simulink library "HybridFEMLibrary"  (Simulink 7.9)
settings: Solver=ode45  SolverMode=SingleTasking  StartTime=0.0  StopTime=10.0  RelTol=1e-3
values from neighbouring files (symbols this model uses):
  Elements = ElementsBack    [ModelSetup.m]
  Integrator = CreateIntegrator(data(3), data(4), data(5), data(1), data(2))    [LoadConfiguration.m]    (also in MatlabSimulation.m = UpdateAccelerationCR(Integrator, Structure, step); ModelSetup.m = InitializeIntegrator(Integrator, Structure))
  sample = SampleRate/Integrator.Interpolations    [ModelSetup.m]
  SampleRate = Integrator.Timestep    [ModelSetup.m]
  Structure = CalculateMatrices(Structure, Elements, Integrator)    [ModelSetup.m]
undefined symbols (not defined in the file or in its folder): DiscIntNeverNeededParam, MNS
libraries: simulink x2
settings Model: Creator=Tommy  LastModifiedBy=Thomas Marullo

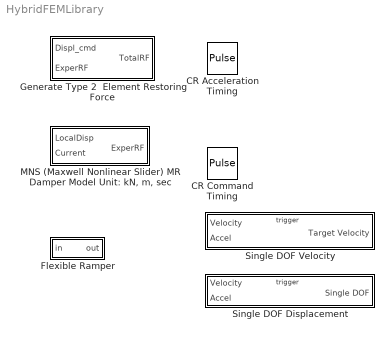
== system HybridFEMLibrary ==
  CR Acceleration Timing : DiscretePulseGenerator  Period=Integrator.Interpolations  PhaseDelay=Integrator.Interpolations-1  SampleTime=sample
  CR Command Timing : DiscretePulseGenerator  Period=Integrator.Interpolations  PulseWidth=Integrator.Interpolations-1  SampleTime=sample
  Flexible Ramper : Subsystem  mask{ramps=Integrator.Interpolations, samplerate=sample, u_old=[0]}
      mask prompts: ramps "Total ramp steps"; samplerate "Sample rate"; u_old "Dimensions"
      mask help:
      | Signal ramper that starts when it detects a change in the current and previous signal. It then ramps for the designated steps and goes back to detecting changes to start ramping again.
      |
      | Set the total number of ramping steps it should interpolate between the current and previous signals.  This will disregard any signal changes for the number of steps desginated.
      | Sample rate should be the sample rate of the system.
      | The source signal sample rate should be the sample rate * total ramp steps to get the best performance.  Otherwise, having a number of ramps smaller than the number of steps between signal changes will result in flat-lining.  Larger ramps than the number of steps between signal changes will result in missed data and poor ramping.
      |
      | Set Dimension variable to an empty array of required size, ie. [0;0;0] for 3 dimensions.
      mask Display:
      | fprintf('%d',ramps)
      | port_label('input',1,'>')
      | port_label('output',1,'>')
  Generate Type 2  Element Restoring Force : Subsystem  mask(Generate Type 2 Element Restoring Force){id=0, simulation=off}
      mask prompts: id "Element ID"; simulation "Experiment Mode"
      mask help:
      | Generates the Restoring Force vector for a Type 2 Element
      |
      | Enter the ID for this element corresponding with the input configuration file.
      |
      | For Simulation mode, uncheck the "Experiment Mode" box.
      | Connect the 'Target Displacement' command from the Integrator to the 'Disp' input.  'ExperRF' is not used with Simulation Mode.
      |
      | For Experiment mode, check the "Experiment Mode" box to activate the Experimental Restoring Force (ExperRF) input.
      | Connect an Experimental Restoring Force feedback (physical or numerical) to the 'ExperRF' input.  The 'Disp' is not used with Experiment mode.
      |
      | Connect the 'TotalRF' output to the 'TotalRF' input of the Integrator block or through a summer block with other Element 'TotalRF' outputs.
      mask Display:
      | disp(id);
      | port_label('input',1,'Disp');
      | port_label('input',2,'ExperRF');
      | port_label('output',1,'TotalRF');
  "MNS (Maxwell Nonlinear Slider) MR Damper Model Unit: kN, m, sec" : Subsystem
      mask Type: MNS MR Damper Model
      mask Description:
      | Used in the local coordinate system, this model requires a Local Displacement from a "Generate Experimental Command" block and feeds the output force to a Type 2 Experimental Element to convert back to global coordinates.
      | 
      | Requires the HybridFEM/scripts/MNS_model_parameters.m file
  Single DOF Displacement : Subsystem  SystemSampleTime=SampleRate  mask{DOF=Elements{1}.Nodes(1).UX}
      mask prompts: DOF "Element DOF"
  Single DOF Velocity : Subsystem  SystemSampleTime=SampleRate  mask{DOF=Elements{1}.Nodes(1).UX}

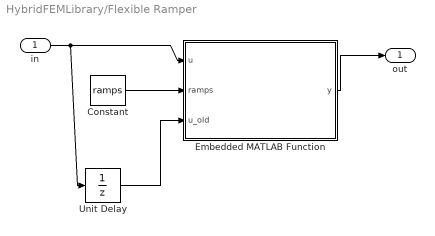
== system HybridFEMLibrary/Flexible Ramper ==
  in : Inport
  Constant : Constant  Value=ramps  SampleTime=samplerate
  Embedded MATLAB Function : MATLAB Function  TreatAsAtomicUnit=on
  Unit Delay : UnitDelay  SampleTime=-1
  out : Outport
  wires:
  in/1 -> Unit Delay/1, Embedded MATLAB Function/1(u)
  Constant/1 -> Embedded MATLAB Function/2(ramps)
  Embedded MATLAB Function/1(y) -> out/1
  Unit Delay/1 -> Embedded MATLAB Function/3(u_old)

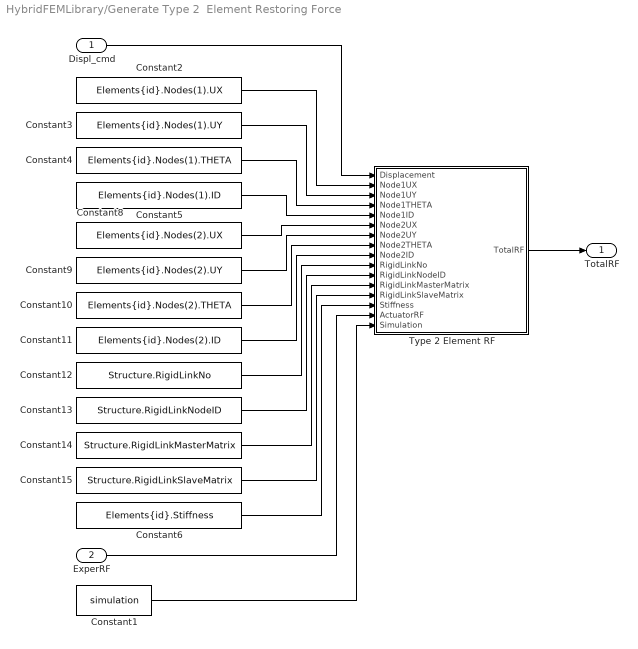
== system HybridFEMLibrary/Generate Type 2  Element Restoring Force ==
  Displ_cmd : Inport
  ExperRF : Inport  Port=2
  Constant1 : Constant  Value=simulation
  Constant10 : Constant  Value=Elements{id}.Nodes(2).THETA
  Constant11 : Constant  Value=Elements{id}.Nodes(2).ID
  Constant12 : Constant  Value=Structure.RigidLinkNo
  Constant13 : Constant  Value=Structure.RigidLinkNodeID
  Constant14 : Constant  Value=Structure.RigidLinkMasterMatrix
  Constant15 : Constant  Value=Structure.RigidLinkSlaveMatrix
  Constant2 : Constant  Value=Elements{id}.Nodes(1).UX
  Constant3 : Constant  Value=Elements{id}.Nodes(1).UY
  Constant4 : Constant  Value=Elements{id}.Nodes(1).THETA
  Constant5 : Constant  Value=Elements{id}.Nodes(1).ID
  Constant6 : Constant  Value=Elements{id}.Stiffness
  Constant8 : Constant  Value=Elements{id}.Nodes(2).UX
  Constant9 : Constant  Value=Elements{id}.Nodes(2).UY
  Type 2 Element RF : MATLAB Function  TreatAsAtomicUnit=on
  TotalRF : Outport
  wires:
  Type 2 Element RF/1(TotalRF) -> TotalRF/1
  Displ_cmd/1 -> Type 2 Element RF/1(Displacement)
  Constant2/1 -> Type 2 Element RF/2(Node1UX)
  Constant3/1 -> Type 2 Element RF/3(Node1UY)
  Constant4/1 -> Type 2 Element RF/4(Node1THETA)
  Constant5/1 -> Type 2 Element RF/5(Node1ID)
  Constant8/1 -> Type 2 Element RF/6(Node2UX)
  Constant9/1 -> Type 2 Element RF/7(Node2UY)
  Constant10/1 -> Type 2 Element RF/8(Node2THETA)
  Constant11/1 -> Type 2 Element RF/9(Node2ID)
  Constant12/1 -> Type 2 Element RF/10(RigidLinkNo)
  Constant13/1 -> Type 2 Element RF/11(RigidLinkNodeID)
  Constant14/1 -> Type 2 Element RF/12(RigidLinkMasterMatrix)
  Constant15/1 -> Type 2 Element RF/13(RigidLinkSlaveMatrix)
  Constant6/1 -> Type 2 Element RF/14(Stiffness)
  ExperRF/1 -> Type 2 Element RF/15(ActuatorRF)
  Constant1/1 -> Type 2 Element RF/16(Simulation)

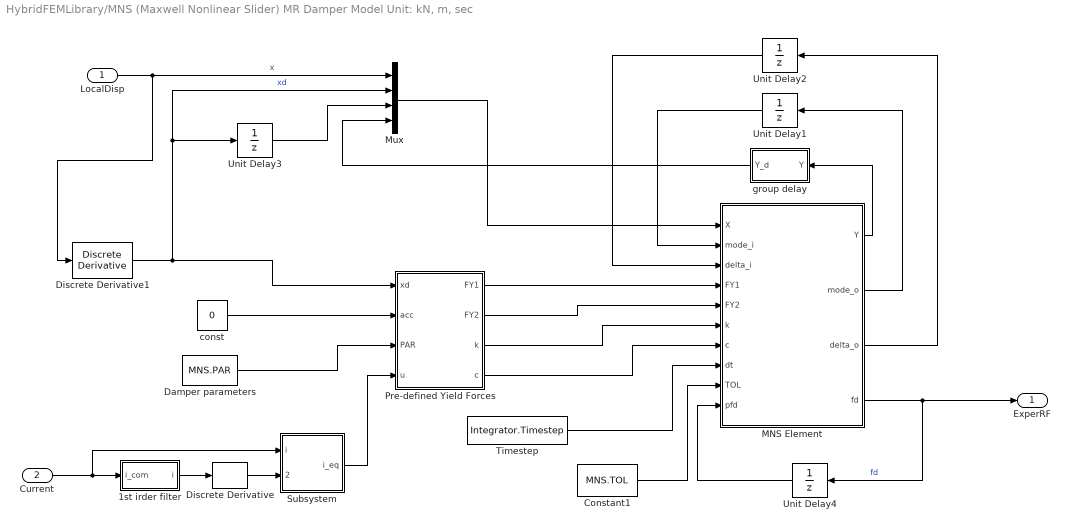
== system HybridFEMLibrary/MNS (Maxwell Nonlinear Slider) MR Damper Model Unit: kN, m, sec ==
  LocalDisp : Inport
  Current : Inport  Port=2
  1st irder filter : Subsystem
  Constant1 : Constant  Value=MNS.TOL
  Damper parameters : Constant  Value=MNS.PAR
  Discrete Derivative : simulink/Discrete/Discrete Derivative  SystemSampleTime=-1  gainval=1.0  ICPrevScaledInput=0.0  OutMin=[]  OutMax=[]  OutDataType=fixdt(1, 16)  OutScaling=2^-10  DoSatur=off
  Discrete Derivative1 : simulink/Discrete/Discrete Derivative  SystemSampleTime=-1  gainval=1.0  ICPrevScaledInput=0.0  OutMin=[]  OutMax=[]  OutDataType=fixdt(1, 16)  OutScaling=2^-10  DoSatur=off
  MNS Element : MATLAB Function  TreatAsAtomicUnit=on
  Mux : Mux
  Pre-defined Yield Forces : MATLAB Function  TreatAsAtomicUnit=on
  Subsystem : Subsystem
  Timestep : Constant  Value=Integrator.Timestep
  Unit Delay{1..4} (4 alike) : UnitDelay  SampleTime=-1
  const : Constant  Value=0
  group delay : Subsystem
  ExperRF : Outport
  wires:
  LocalDisp/1 -> Discrete Derivative1/1, Mux/1  "x"
  Discrete Derivative1/1 -> Mux/2, Unit Delay3/1, Pre-defined Yield Forces/1(xd)  "xd"
  Mux/1 -> MNS Element/1(X)
  MNS Element/4(fd) -> Unit Delay4/1, ExperRF/1  "fd"
  MNS Element/2(mode_o) -> Unit Delay1/1
  Timestep/1 -> MNS Element/8(dt)
  MNS Element/1(Y) -> group delay/1(Y)
  MNS Element/3(delta_o) -> Unit Delay2/1
  Unit Delay2/1 -> MNS Element/3(delta_i)
  Unit Delay1/1 -> MNS Element/2(mode_i)
  group delay/1(Y_d) -> Mux/4
  Unit Delay3/1 -> Mux/3
  Damper parameters/1 -> Pre-defined Yield Forces/3(PAR)
  Constant1/1 -> MNS Element/9(TOL)
  Unit Delay4/1 -> MNS Element/10(pfd)
  Pre-defined Yield Forces/3(k) -> MNS Element/6(k)
  Pre-defined Yield Forces/4(c) -> MNS Element/7(c)
  Current/1 -> Subsystem/1(i), 1st irder filter/1(i_com)
  Pre-defined Yield Forces/1(FY1) -> MNS Element/4(FY1)
  Pre-defined Yield Forces/2(FY2) -> MNS Element/5(FY2)
  Subsystem/1(i_eq) -> Pre-defined Yield Forces/4(u)
  Discrete Derivative/1 -> Subsystem/2(i_eq_dot)
  const/1 -> Pre-defined Yield Forces/2(acc)
  1st irder filter/1(i) -> Discrete Derivative/1

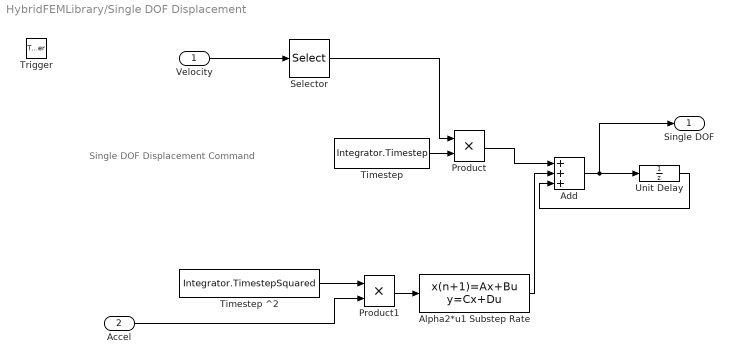
== system HybridFEMLibrary/Single DOF Displacement ==
  note: Single DOF Displacement Command
  Velocity : Inport
  Accel : Inport  Port=2
  Trigger : TriggerPort
  Add : Sum  Inputs=+++
  Alpha2*u1 Substep Rate : DiscreteStateSpace  A=[]  B=[]  C=[]  D=Integrator.Alpha2(DOF,:)  SampleTime=-1
  Product : Product  RndMeth=Zero
  Product1 : Product  RndMeth=Zero
  Selector : Selector  InputPortWidth=NumFreeDOF  IndexOptions=Index vector (dialog)  Indices=DOF  OutputSizes=1
  Timestep : Constant  Value=Integrator.Timestep
  Timestep ^2 : Constant  Value=Integrator.TimestepSquared
  Unit Delay : UnitDelay  SampleTime=-1
  Single DOF : Outport
  wires:
  Unit Delay/1 -> Add/3
  Alpha2*u1 Substep Rate/1 -> Add/2
  Selector/1 -> Product/1
  Velocity/1 -> Selector/1
  Add/1 -> Unit Delay/1, Single DOF/1
  Product1/1 -> Alpha2*u1 Substep Rate/1
  Accel/1 -> Product1/2
  Timestep ^2/1 -> Product1/1
  Timestep/1 -> Product/2
  Product/1 -> Add/1

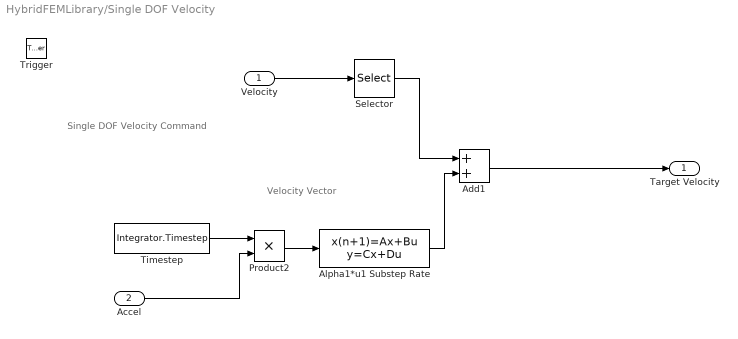
== system HybridFEMLibrary/Single DOF Velocity ==
  note: Velocity Vector
  note: Single DOF Velocity Command
  Velocity : Inport
  Accel : Inport  Port=2
  Trigger : TriggerPort
  Add1 : Sum
  Alpha1*u1 Substep Rate : DiscreteStateSpace  A=[]  B=[]  C=[]  D=Integrator.Alpha1(DOF,:)  SampleTime=-1
  Product2 : Product  RndMeth=Zero
  Selector : Selector  InputPortWidth=NumFreeDOF  IndexOptions=Index vector (dialog)  Indices=DOF  OutputSizes=1
  "Timestep " : Constant  Value=Integrator.Timestep
  Target Velocity : Outport
  wires:
  Selector/1 -> Add1/1
  Accel/1 -> Product2/2
  Product2/1 -> Alpha1*u1 Substep Rate/1
  "Timestep "/1 -> Product2/1
  Alpha1*u1 Substep Rate/1 -> Add1/2
  Add1/1 -> Target Velocity/1
  Velocity/1 -> Selector/1

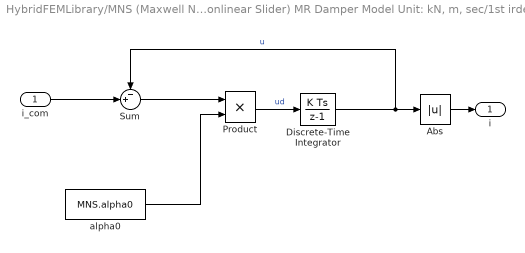
== system HybridFEMLibrary/MNS (Maxwell Nonlinear Slider) MR Damper Model Unit: kN, m, sec/1st irder filter ==
  i_com : Inport
  Abs : Abs
  Discrete-Time Integrator : DiscreteIntegrator  SampleTime=-1  ICPrevOutput=DiscIntNeverNeededParam  ICPrevScaledInput=DiscIntNeverNeededParam
  Product : Product  RndMeth=Zero
  Sum : Sum  Inputs=-+|
  alpha0 : Constant  Value=MNS.alpha0
  i : Outport
  wires:
  Abs/1 -> i/1
  alpha0/1 -> Product/2
  Sum/1 -> Product/1
  i_com/1 -> Sum/2
  Discrete-Time Integrator/1 -> Abs/1, Sum/1  "u"
  Product/1 -> Discrete-Time Integrator/1  "ud"

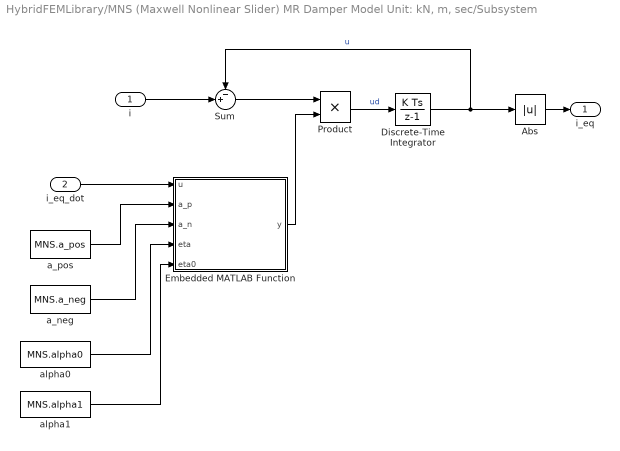
== system HybridFEMLibrary/MNS (Maxwell Nonlinear Slider) MR Damper Model Unit: kN, m, sec/Subsystem ==
  i : Inport
  i_eq_dot : Inport  Port=2
  Abs : Abs
  Discrete-Time Integrator : DiscreteIntegrator  SampleTime=-1  ICPrevOutput=DiscIntNeverNeededParam  ICPrevScaledInput=DiscIntNeverNeededParam
  Embedded MATLAB Function : MATLAB Function  TreatAsAtomicUnit=on
  Product : Product  RndMeth=Zero
  Sum : Sum  Inputs=-+|
  a_neg : Constant  Value=MNS.a_neg
  a_pos : Constant  Value=MNS.a_pos
  alpha0 : Constant  Value=MNS.alpha0
  alpha1 : Constant  Value=MNS.alpha1
  i_eq : Outport
  wires:
  i_eq_dot/1 -> Embedded MATLAB Function/1(u)
  a_pos/1 -> Embedded MATLAB Function/2(a_p)
  Product/1 -> Discrete-Time Integrator/1  "ud"
  Discrete-Time Integrator/1 -> Sum/1, Abs/1  "u"
  i/1 -> Sum/2
  Sum/1 -> Product/1
  Embedded MATLAB Function/1(y) -> Product/2
  Abs/1 -> i_eq/1
  alpha0/1 -> Embedded MATLAB Function/4(eta)
  a_neg/1 -> Embedded MATLAB Function/3(a_n)
  alpha1/1 -> Embedded MATLAB Function/5(eta0)

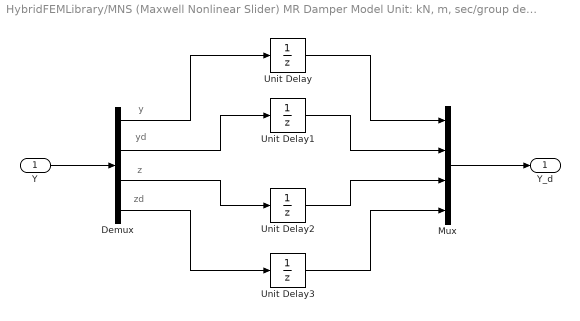
== system HybridFEMLibrary/MNS (Maxwell Nonlinear Slider) MR Damper Model Unit: kN, m, sec/group delay ==
  note: y
  note: yd
  note: z
  note: zd
  Y : Inport
  Demux : Demux
  Mux : Mux
  Unit Delay : UnitDelay  X0=MNS.y0  SampleTime=-1
  Unit Delay1 : UnitDelay  X0=MNS.yd0  SampleTime=-1
  Unit Delay2 : UnitDelay  X0=MNS.z0  SampleTime=-1
  Unit Delay3 : UnitDelay  X0=MNS.zd0  SampleTime=-1
  Y_d : Outport
  wires:
  Y/1 -> Demux/1
  Unit Delay/1 -> Mux/1
  Demux/2 -> Unit Delay1/1
  Unit Delay1/1 -> Mux/2
  Mux/1 -> Y_d/1
  Demux/3 -> Unit Delay2/1
  Unit Delay2/1 -> Mux/3
  Demux/4 -> Unit Delay3/1
  Unit Delay3/1 -> Mux/4
  Demux/1 -> Unit Delay/1

== matlab function Generate Type 2 Element Restoring Force/Type 2 Element RF ==
  data: NumFreeDOF parameter double; Displacement input double; TotalRF output double; Node1UX input double; Node1UY input double; Node1THETA input double; Node1ID input double; Node2UX input double; Node2UY input double; Node2THETA input double; Node2ID input double; RigidLinkNo input double; RigidLinkNodeID input double; RigidLinkMasterMatrix input double; RigidLinkSlaveMatrix input double; Stiffness input double; ActuatorRF input double; Simulation input double
% Get restoring force for the element
% Returns (6x1) restoring force vector of element in global coordinates
function TotalRF  = eml(NumFreeDOF, Displacement, ...                        
                        Node1UX, ...
                        Node1UY, ...
                        Node1THETA, ...
                        Node1ID, ...                        
                        Node2UX, ...
                        Node2UY, ...
                        Node2THETA, ...
                        Node2ID, ...
                        RigidLinkNo, ...
                        RigidLinkNodeID, ...
                        RigidLinkMasterMatrix, ...
                        RigidLinkSlaveMatrix, ...  
                        Stiffness, ...
                        ActuatorRF, ... 
                        Simulation)              

% Persistent variables to remain in memory

% Initialize the persistent variables

% Create the displacement (6x1) vector of the element in global coordinates
    Ue=zeros(6,1);
    dof=zeros(6,1);
    dof(1,1)=Node1UX;
    dof(2,1)=Node1UY;
    dof(3,1)=Node1THETA;
    dof(4,1)=Node2UX;
    dof(5,1)=Node2UY;
    dof(6,1)=Node2THETA;
    for i=1:6
        if dof(i,1) ~= -1
            Ue(i,1)=Displacement(dof(i,1),1);
        end
    end

% Check if it is a simulation or using real restoring force
SE = zeros(6,6);
if (Simulation == 0)    
    % Form Stiffness Matrix
    SE(1, 1) = Stiffness;
    SE(1, 4) = -Stiffness;
    SE(4, 4) = Stiffness;
    SE(4, 1) = SE(1,4);
        
    RestoringForce = SE*Ue;  % Resisting (6x1) force vector of element in global coordinates
else        
    RestoringForce = zeros(6,1);
    RestoringForce(1,1) = ActuatorRF;
    RestoringForce(4,1) = -ActuatorRF;
end

% Rigid Link Calculations
TR = eye(6,6); % Transformation matrix for rigid link
if( RigidLinkNo )    
    % Find the row with the slave node, if it exists in the element
    idx = 0;
    for kk = 1:RigidLinkNo
        if (RigidLinkNodeID(2,kk) == Node1ID)
            idx = kk;
            break;
        end
    end
    %idx=find(RigidLinkNodeID(2,:) == Node1ID); % find if a slave node exists in the element
    if ( idx )
        TL=Calculate_RigidLink_Transformation(RigidLinkMasterMatrix(2,idx),RigidLinkMasterMatrix(3,idx),RigidLinkSlaveMatrix(2,idx),RigidLinkSlaveMatrix(3,idx));
        jjj = 1; % Node 1
        TR(3*(jjj-1)+1:3*jjj,3*(jjj-1)+1:3*jjj) = TL;
    end
    idx = 0;
    for kk = 1:RigidLinkNo
        if (RigidLinkNodeID(2,kk) == Node2ID)
            idx = kk;
            break;
        end
    end    
    %idx=find(RigidLinkNodeID(2,:) == Node2ID); % find if a slave node exists in the element
    if ( idx )
        TL=Calculate_RigidLink_Transformation(RigidLinkMasterMatrix(2,idx),RigidLinkMasterMatrix(3,idx),RigidLinkSlaveMatrix(2,idx),RigidLinkSlaveMatrix(3,idx));
        jjj = 2; % Node 2
        TR(3*(jjj-1)+1:3*jjj,3*(jjj-1)+1:3*jjj) = TL;
    end    
    
    Ue = TR * Ue;  
    RestoringForce = TR' * SE * Ue;  
end

% Form total restoring force vector
TotalRF = zeros(NumFreeDOF, 1);
    
% Get element nodes to assemble in the structure restoring force vector
if Node1UX ~= -1
    TotalRF(Node1UX, 1) = RestoringForce(1, 1);
end
if Node1UY ~= -1
    TotalRF(Node1UY, 1) = RestoringForce(2, 1);
end
if Node1THETA ~= -1
    TotalRF(Node1THETA, 1) = RestoringForce(3, 1);
end
if Node2UX ~= -1
    TotalRF(Node2UX, 1) = RestoringForce(4, 1);
end
if Node2UY ~= -1
    TotalRF(Node2UY, 1) = RestoringForce(5, 1);
end
if Node2THETA ~= -1
    TotalRF(Node2THETA, 1) = RestoringForce(6, 1);
end

% Calculate Rigid Link Transformation
function TL = Calculate_RigidLink_Transformation(MNXcoord, MNYcoord, SNXcoord, SNYcoord)
X1 = MNXcoord; Y1 = MNYcoord;
X2 = SNXcoord;  Y2 = SNYcoord;
deltaX = X2 - X1;
deltaY = Y2 - Y1;
TL = [ 1 0 -deltaY;
       0 1  deltaX;
       0 0  1    ];

== matlab function Flexible Ramper/Embedded MATLAB Function ==
  data: u input double; y output double; ramps input double; u_old input double
function y  = fcn(u,ramps,u_old)
 
% persistent delay_count;
% 
% if isempty(delay_count)
%     delay_count = 0;
% end
% 
% if delay_count < delay
%     delay_count = delay_count + 1;
%     y = u;
%     rampstep_out = 1;
%     u_old_out = u;
% else
% 

persistent isRamping;
persistent startPoint;
persistent endPoint;
persistent rampstep;

if isempty(isRamping)
    isRamping = 0;    
    startPoint = 0;
    endPoint = 0;
    rampstep = 0;
end

%% Check if u and u_old
if (u == u_old && ~isRamping);
    % Do nothing and hold here    
    y = u;
elseif isRamping ;
    % Do nothing
    y = u;
else
    isRamping = 1; % Start first ramping
    startPoint = u_old; % get values
    endPoint = u; % get values    
    rampstep = 1;     
end

% Ramp process
if isRamping      
    y = (endPoint - startPoint)/ramps * rampstep + startPoint;  
    if (rampstep == ramps)
        isRamping = 0;
    else
        rampstep = rampstep + 1;
    end 
else
    y = u;
end


    

%% Ramp
% y = (u - u_old)/ramps * rampstep + u_old;    
%     
% %% Reset ramper
% if (rampstep == ramps)
%     rampstep_out = 1;
%     u_old_out = u; %save this displacement for the base of the next ramped command
% else
%     rampstep_out = rampstep + 1;
%     u_old_out = u_old;
% end
%     
% end

== matlab function MNS (Maxwell Nonlinear Slider) MR Damper Model Unit: kN, m, sec/Subsystem/Embedded MATLAB Function ==
  data: u input double; y output double; a_p input double; a_n input double; eta input double; eta0 input double
function y = fcn(u,a_p,a_n,eta,eta0)
% This block supports the Embedded MATLAB subset.
% See the help menu for details. 

if( u < 0 )
    y = a_n*abs(u)^1 + eta0;    
else
    y = a_p*abs(u) + eta0;
end

== matlab function MNS (Maxwell Nonlinear Slider) MR Damper Model Unit: kN, m, sec/MNS Element ==
  data: X input double; mode_i input double; delta_i input double; FY1 input double; FY2 input double; Y output double; mode_o output double; delta_o output double; fd output double; k input double; c input double; dt input double; TOL input double; pfd input double
function [Y,mode_o,delta_o,fd] = NL_maxwell(X,mode_i,delta_i,FY1,FY2,k,c,dt,TOL,pfd)
% X = [x xd y yd z zd]' : state vector
% Y = [y yd z zd]'

Y=zeros(4,1);
mode_o = mode_i;
delta_o = delta_i;
fd = FY1;

x = X(1);   xd = X(2);  xd_p = X(3);
y = X(4);   yd = X(5);
z = X(6);   zd = X(7);

if( mode_i == 0 )    % stick mode (pre-yield mode)

    y = x - delta_i;
    yd = xd;
    
    zd = k/c*(y-z);
    z = z + zd*dt;
    
    fd = k*(y-z);
    delta_fd = fd - pfd;
    
    if( (FY1 - fd)*(FY2 - fd) > 0 )
        if( delta_fd > 0 )
            if( fd - FY1 > TOL )
                fd = FY1;
                mode_i = 1;  
            end
        else
            if( FY2-fd > TOL )
                fd = FY2;
                mode_i = 2;  
            end
        end
    end
    
    mode_o = mode_i;        
    delta_o = delta_i;

end 

if( mode_i > 0 )   % slide mode (post-yield mode)
    
    if( mode_i == 1)
        fd = FY1;
    else
        fd = FY2;
    end
       
    zd = fd/c;
    z = z + zd*dt;
    y2 = fd/k + z;
    yd2 = (y2 - y)/dt;
    y=y2;
    
    if( (xd - yd2)*(xd_p - yd) < 0 ) % check mode change
        mode_o = 0;          
        delta_o = x - y;
    end
    
    yd = yd2;
    
end

%%%%
if( FY1 == FY2 )
    if( fd > 0 )
        mode_o = 1;
    else
        mode_o = 2;
    end
end
%%%%
Y = [y yd z zd]';

== matlab function MNS (Maxwell Nonlinear Slider) MR Damper Model Unit: kN, m, sec/Pre-defined Yield Forces ==
  data: xd input double; acc input double; PAR input double; u input double; FY1 output double; FY2 output double; k output double; c output double
function [FY1,FY2, k, c] = fcn(xd,acc,PAR,u)
% PAR columns
% 1:current  2:c  3:k  4:vm  5:vcr1  6:vcr2
% 7:a1  8:a2  9:a3  10:a4  11:a5  12:a6
% vm : virtual mass to describe the force drop of post-yield curve
% vcr : velocity from which the post yield curve is considered as linear


[in l2]=size(PAR);
I1=1; I2=1;
% searching for interpolation
for i=1:in-1
    if( u >= PAR(i,1) && u < PAR(i+1,1) )
        I1=i; I2=i+1;
    end
end

% calculate proportional ratio of input current
r= (u - PAR(I1,1)) / (PAR(I2,1) - PAR(I1,1));

par = PAR(I1,:) + r*(PAR(I2,:) - PAR(I1,:));

c=par(2); k=par(3); vm=par(4); vcr1=par(5); vcr2=par(6);
a1=par(7); a2=par(8); a3=par(9); a4=par(10); a5=par(11); a6=par(12);

%% Herschel-Bulkley visco-plasticity model
fcr1 = a1+a2*vcr1^a3; 
fcr2 = a4+a5*abs(vcr2)^a6; 

if( xd >= vcr1 )
    FY1 = a1+a2*abs(xd)^a3;
else
    ap = a2*a3*abs(vcr1)^(a3-1);
    FY1 = ap*(xd-vcr1)+fcr1;
end
    
if( xd < vcr2 )
    FY2 = a4+a5*abs(xd)^a6;
else
    ap = -a5*a6*abs(vcr2)^(a6-1); 
    FY2 = ap*(xd-vcr2)+fcr2;
end


if( acc < 0 )
    FY1 = FY1 + vm*acc;
end

if( acc > 0 )
    FY2 = FY2 + vm*acc;
end
